simulink model "simulateur_final"  (R2019a)
settings: Solver=FixedStepAuto  StartTime=0.0  StopTime=1  FixedStep=0.01  RelTol=1e-3
model workspace (MAT data in the model file):
  lame = Simulink.Signal
  lame.DataType = 'auto'
  lame.Dimensions = -1
  lame.DimensionsMode = 'auto'
  lame.Complexity = 'auto'
  lame.SampleTime = -1
  lame.SamplingMode = 'auto'
libraries: simulink x1
settings Model: Creator=phant  LastModifiedBy=phant
settings SolverCC: AlgebraicLoopSolver=LineSearch

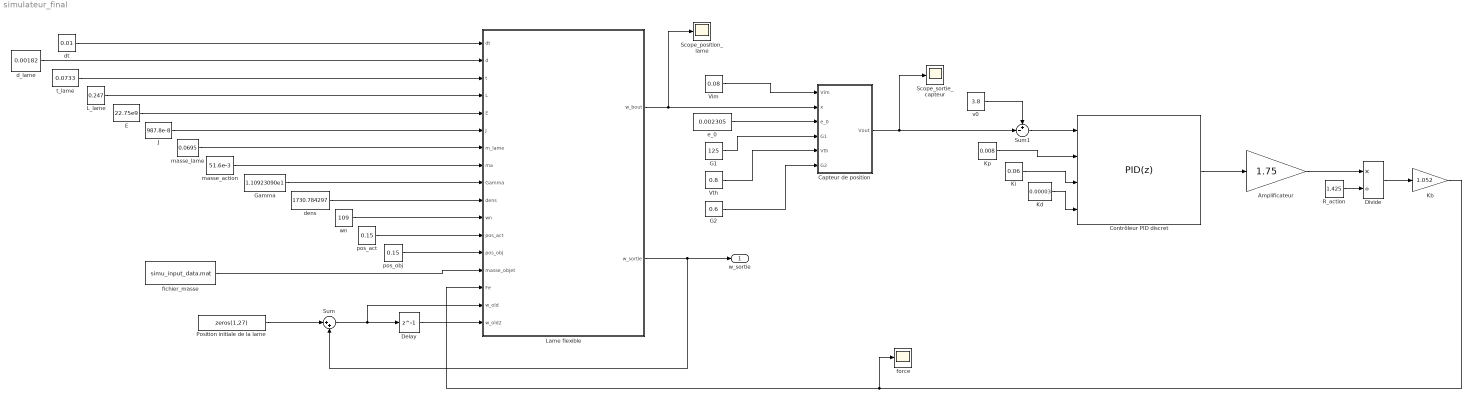
== system simulateur_final ==
  Amplificateur : Gain  Gain=1.75
  Capteur de position : MATLAB Function  TreatAsAtomicUnit=on
  Contrôleur PID discret : simulink/Continuous/PID Controller  Controller=PID  Form=Parallel  TimeDomain=Discrete-time  SampleTime=-1  IntegratorMethod=Forward Euler  FilterMethod=Forward Euler  ControllerParametersSource=external  P=0.008  I=0.06  D=0.00003  UseFilter=off  N=100  TunerSelectOption=Transfer Function Based (PID Tuner App)  InitialConditionSource=internal  InitialConditionForIntegrator=0  InitialConditionForFilter=0  DifferentiatorICPrevScaledInput=0  ExternalReset=none  TrackingMode=off  Kt=1  LimitOutput=off  UpperSaturationLimit=inf  LowerSaturationLimit=-inf  LinearizeAsGain=off  AntiWindupMode=none  Kb=1  POutMin=[]  POutMax=[]  IOutMin=[]  IOutMax=[]  DOutMin=[]  DOutMax=[]  NOutMin=[]  NOutMax=[]  SumOutMin=[]  SumOutMax=[]  SaturationOutMin=[]  SaturationOutMax=[]  PParamMin=[]  PParamMax=[]  IParamMin=[]  IParamMax=[]  DParamMin=[]  DParamMax=[]  NParamMin=[]  NParamMax=[]  KbParamMin=[]  KbParamMax=[]  KtParamMin=[]  KtParamMax=[]  KbOutMin=[]  KbOutMax=[]  KtOutMin=[]  KtOutMax=[]  IntegratorOutMin=[]  IntegratorOutMax=[]  FilterOutMin=[]  FilterOutMax=[]  SumI1OutMin=[]  SumI1OutMax=[]  SumI2OutMin=[]  SumI2OutMax=[]  SumI3OutMin=[]  SumI3OutMax=[]  SumI4OutMin=[]  SumI4OutMax=[]  SumDOutMin=[]  SumDOutMax=[]  DifferentiatorOutMin=[]  DifferentiatorOutMax=[]  FilterDiffOutCoefMin=[]  FilterDiffOutCoefMax=[]  ReciprocalOutMin=[]  ReciprocalOutMax=[]  SumDenOutMin=[]  SumDenOutMax=[]  SumNumOutMin=[]  SumNumOutMax=[]  DivideOutMin=[]  DivideOutMax=[]  IntegratorContinuousStateAttributes=''  IntegratorStateMustResolveToSignalObject=off  IntegratorRTWStateStorageClass=Auto  FilterContinuousStateAttributes=''  FilterStateMustResolveToSignalObject=off  FilterRTWStateStorageClass=Auto  ParallelPVariant=ExternalParameters  IdealPVariant=Disabled  IVariant=ExternalParameters  DVariant=ExternalParameters  IntegratorVariant=Discrete  SatVariant=Disabled  AWVariant=Passthrough  PCopyVariant=Disabled  TRVariant=Disabled  FdbkBlocksVariant=Forward  IdealPFdbkVariant=Disabled  SatFdbkVariant=Disabled  DerivativeFilterVariant=Differentiator  NVariant=Passthrough  NCopyVariant=Disabled_SignalSpec  FilterICVariant=InternalICsDifferentiator  IntegratorICVariant=InternalICs  ExternalResetVariant=Disabled  TRSumVariant=Passthrough  SumFdbkVariant=Disabled  SumVariant=Sum_PID
  Delay : Delay  DelayLength=1  InitialCondition=0
  Divide : Product  Inputs=*/
  E : Constant  Value=22.75e9
  G1 : Constant  Value=125
  G2 : Constant  Value=0.6
  Gamma : Constant  Value=1.10923090e1
  J : Constant  Value=987.8e-8
  Kb : Gain  Gain=1.052
  Kd : Constant  Value=0.00003
  Ki : Constant  Value=0.06
  Kp : Constant  Value=0.008
  L_lame : Constant  Value=0.247
  Lame flexible : MATLAB Function  TreatAsAtomicUnit=on
  Position initiale de la lame : Constant  Value=zeros(1,27)  VectorParams1D=off
  R_action : Constant  Value=1.425
  Scope_position_lame : Scope
  Scope_sortie_capteur : Scope
  Sum : Sum  Inputs=|++
  Sum1 : Sum  Inputs=+-|
  Vim : Constant  Value=0.08
  Vth : Constant  Value=0.8
  d_lame : Constant  Value=0.00182
  dens : Constant  Value=1730.784297
  dt : Constant  Value=0.01
  e_0 : Constant  Value=0.002305
  fichier_masse : FromFile  FileName=simu_input_data.mat  SampleTime=0
  force : Scope
  masse_action : Constant  Value=51.6e-3
  masse_lame : Constant  Value=0.0695
  pos_act : Constant  Value=0.15
  pos_obj : Constant  Value=0.15
  t_lame : Constant  Value=0.0733
  v0 : Constant  Value=3.8
  wn : Constant  Value=109
  w_sortie : Outport
  wires:
  G2/1 -> Capteur de position/6(G2)
  Vth/1 -> Capteur de position/5(Vth)
  G1/1 -> Capteur de position/4(G1)
  Vim/1 -> Capteur de position/1(Vim)
  e_0/1 -> Capteur de position/3(e_0)
  Contrôleur PID discret/1 -> Amplificateur/1
  pos_act/1 -> Lame flexible/12(pos_act)
  Gamma/1 -> Lame flexible/9(Gamma)
  E/1 -> Lame flexible/5(E)
  J/1 -> Lame flexible/6(J)
  L_lame/1 -> Lame flexible/4(L)
  masse_lame/1 -> Lame flexible/7(m_lame)
  wn/1 -> Lame flexible/11(wn)
  masse_action/1 -> Lame flexible/8(ma)
  t_lame/1 -> Lame flexible/3(t)
  d_lame/1 -> Lame flexible/2(d)
  dens/1 -> Lame flexible/10(dens)
  Lame flexible/1(w_bout) -> Scope_position_lame/1, Capteur de position/2(x)
  dt/1 -> Lame flexible/1(dt)
  Kp/1 -> Contrôleur PID discret/2
  Ki/1 -> Contrôleur PID discret/3
  Kd/1 -> Contrôleur PID discret/4
  Amplificateur/1 -> Divide/1
  Kb/1 -> force/1, Lame flexible/15(Fe)
  R_action/1 -> Divide/2
  Divide/1 -> Kb/1
  Capteur de position/1(Vout) -> Scope_sortie_capteur/1, Sum1/2
  Sum1/1 -> Contrôleur PID discret/1
  v0/1 -> Sum1/1
  pos_obj/1 -> Lame flexible/13(pos_obj)
  Lame flexible/2(w_sortie) -> w_sortie/1, Sum/2
  Position initiale de la lame/1 -> Sum/1
  Sum/1 -> Lame flexible/16(w_old), Delay/1
  Delay/1 -> Lame flexible/17(w_old2)
  fichier_masse/1 -> Lame flexible/14(masse_objet)

== matlab function simulateur_final/Capteur de position ==
  data: Vim input; Vout output; x input; e_0 input; G1 input; Vth input; G2 input
function Vout = fcn(Vim,x,e_0,G1,Vth,G2)

Vout = ((Vim/2)*(1+x/e_0)*G1 - Vth)*G2;

== matlab function simulateur_final/Lame flexible ==
  data: dt input; d input; t input; L input; E input; J input; m_lame input; ma input; Gamma input; dens input; wn input; pos_act input; pos_obj input; masse_objet input; Fe input; w_bout output; w_old input size=[1,27]; w_old2 input size=[1,27]; w_sortie output size=[1,27]
function [w_bout,w_sortie] = pos_lame(dt, d, t, L, E, J, m_lame, ma, Gamma, dens, wn, pos_act, pos_obj, masse_objet, Fe, w_old, w_old2)
%     dens = m_lame/(L*t*d);
%     m_lame = dens*d*t*L;
    mu =  m_lame/L;
%     mu = dens*d*t; % Masse linÃ©ique kg/m 
%     E = ((wn^2)*mu*(L^4))/((1.8751^4)*J);
    nx = 25;         % Nb d'Ã©lÃ©ments spatiaux
    
    dx =   L/(nx-1); % incrÃ©ment spatial
    x  = -dx:dx:L+dx;     % grille spatiale
    nx = nx+2;
    
    m = masse_objet+ma+mu*L;
    amo = -Gamma*m;
    
    index_obj = round((pos_obj/L)*nx);
    index_act = round((pos_act/L)*nx);

    %% Vecteur qui condiendra la position de l'extrÃ©mitÃ© de la lame en fonction
    % du temps
    w_bout = 0;

    %% PrÃ©calcul des params de simulation pour accÃ©lerer la boucle
    coeff1 = ((6*E*J*(dt^2)/((dx^4)*(amo*dt-mu)))-((2*mu)/(amo*dt-mu))+((amo*dt)/(amo*dt-mu)));
    coeff2 = ((4*E*J*dt^2)/((dx^4)*(amo*dt-mu)));
    coeff3 = ((E*J*(dt^2))/((dx^4)*(amo*dt-mu)));
    coeff4 = ((mu)/(amo*dt-mu));
    coeff5 = ((dt^2)/(dx*(amo*dt-mu)));

    Fo = masse_objet * (-9.81); %Force de l'objet ajoute
    Fa = ma * (-9.81); %Force actionneur

    Fp = m_lame*(-9.81);
    vecteur_objet = zeros(1,nx);
    vecteur_objet(index_obj) = Fo;
    vecteur_actionneur = zeros(1,nx);
    vecteur_actionneur(index_act) = Fa + Fe;
    Hum = ones(1,nx);
    vecteur_poutre = (Fp/nx)*Hum;
    vecteur_forces = zeros(1,nx);
    vecteur_forces = vecteur_objet + vecteur_actionneur + vecteur_poutre;

    i = 3:nx-2;
    w_sortie = zeros(1,nx);
    w_sortie(i) = (coeff1*w_old(i)-coeff2*(w_old(i+1)+w_old(i-1))+coeff3*(w_old(i+2)+w_old(i-2))+w_old2(i)*coeff4-coeff5*(vecteur_forces(i)));
    %% Conditions limites 
    w_sortie(1:2) = 0;                 % ClampÃ© Ã  zero, position et dÃ©rivÃ©e nulle

    w_sortie(end-1) = 2*w_sortie(end-2)-w_sortie(end-3);    % Libre au bout dÃ©rivÃ©es 2e et 3e nulles
    w_sortie(end) = 2*w_sortie(end-1)-w_sortie(end-2);

    w_bout = w_sortie(end);
end
